simulink model "cIPC_l2originalLoad"  (R2024b)
settings: Solver=FixedStepDiscrete  StartTime=0.0  StopTime=TMax  FixedStep=DT  RelTol=1e-3
undefined symbols (not defined in the file): DiscIntNeverNeededParam, DT, Ki, optimal_azimuth_offset_rad
libraries: simulink_extras x1
settings Model: Creator=jhummel  LastModifiedBy=jhummel
settings ModelReferenceCC: EnableRefExpFcnMdlSchedulingChecks=on
settings RTWCC: GPUComputeCapability=3.5

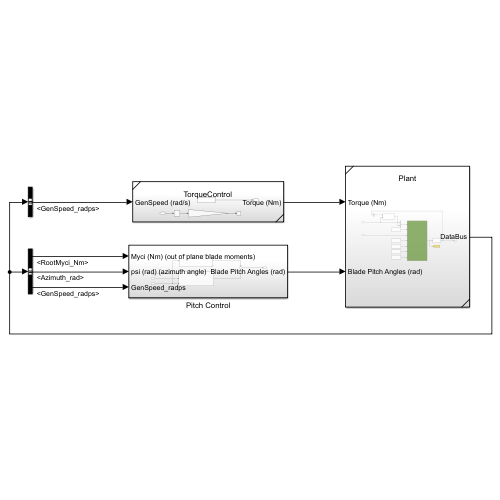
[thumbnail: Simulink's stored preview of the top-level diagram]
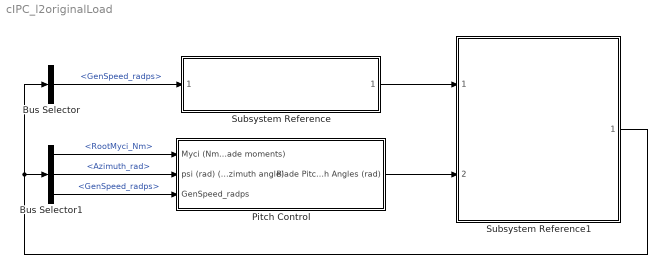
== system cIPC_l2originalLoad ==
  Bus Selector : BusSelector  OutputSignals=GenSpeed_radps
  Bus Selector1 : BusSelector  OutputSignals=RootMyci_Nm,Azimuth_rad,GenSpeed_radps
  Pitch Control : Subsystem
  Subsystem Reference : Subsystem  ReferencedSubsystem=TorqueControl
  Subsystem Reference1 : Subsystem  ReferencedSubsystem=Plant
  wires:
  Bus Selector/1 -> Subsystem Reference/1  "<GenSpeed_radps>"
  Bus Selector1/1 -> Pitch Control/1(Myci (Nm) (out of plane blade moments))  "<RootMyci_Nm>"
  Bus Selector1/2 -> Pitch Control/2(psi (rad) (azimuth angle))  "<Azimuth_rad>"
  Bus Selector1/3 -> Pitch Control/3(GenSpeed_radps)  "<GenSpeed_radps>"
  Subsystem Reference1/1 -> Bus Selector/1, Bus Selector1/1
  Pitch Control/1(Blade Pitch Angles (rad)) -> Subsystem Reference1/2
  Subsystem Reference/1 -> Subsystem Reference1/1

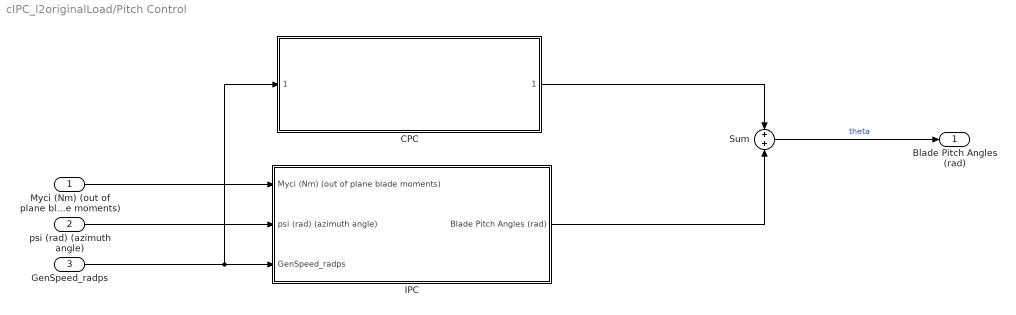
== system cIPC_l2originalLoad/Pitch Control ==
  Myci (Nm) (out of plane blade moments) : Inport
  psi (rad) (azimuth angle) : Inport  Port=2
  GenSpeed_radps : Inport  Port=3
  CPC : Subsystem  ReferencedSubsystem=CollectivePitchControl
  IPC : Subsystem
  Sum : Sum  Inputs=+|+
  Blade Pitch Angles (rad) : Outport
  wires:
  Myci (Nm) (out of plane blade moments)/1 -> IPC/1(Myci (Nm) (out of plane blade moments))
  psi (rad) (azimuth angle)/1 -> IPC/2(psi (rad) (azimuth angle))
  GenSpeed_radps/1 -> CPC/1, IPC/3(GenSpeed_radps)
  CPC/1 -> Sum/1
  Sum/1 -> Blade Pitch Angles (rad)/1  "theta"
  IPC/1(Blade Pitch Angles (rad)) -> Sum/2

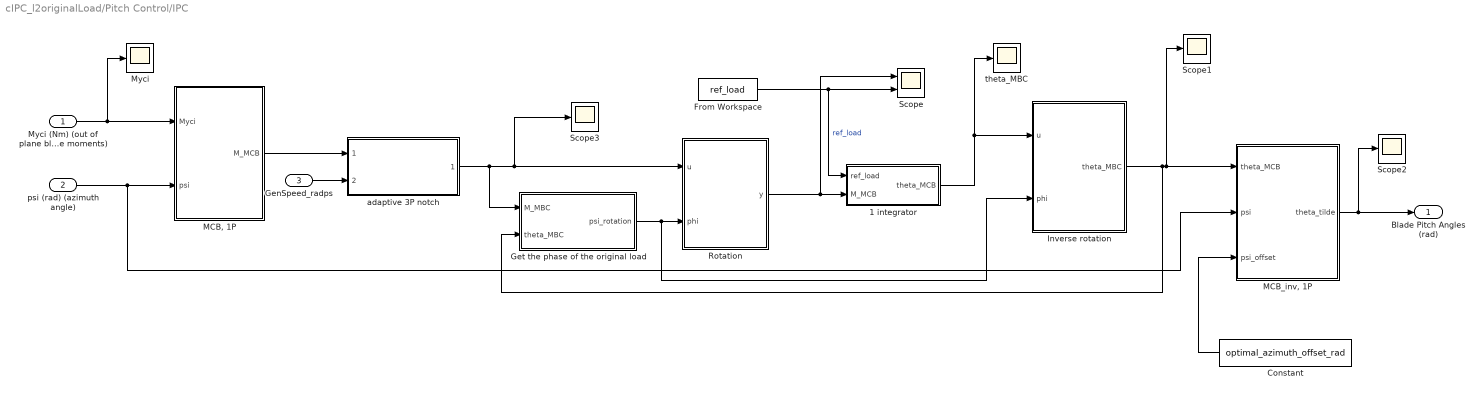
== system cIPC_l2originalLoad/Pitch Control/IPC ==
  Myci (Nm) (out of plane blade moments) : Inport
  psi (rad) (azimuth angle) : Inport  Port=2
  GenSpeed_radps : Inport  Port=3
  1 integrator : Subsystem
  Constant : Constant  Value=optimal_azimuth_offset_rad
  From Workspace : FromWorkspace  VariableName=ref_load  SampleTime=DT
  Get the phase of the original load : Subsystem
  Inverse rotation : Subsystem
  "MCB, 1P" : MATLAB Function  TreatAsAtomicUnit=on
  "MCB_inv, 1P" : MATLAB Function  TreatAsAtomicUnit=on
  Myci : Scope
  Rotation : MATLAB Function  TreatAsAtomicUnit=on
  Scope : Scope  NumInputPorts=2
  Scope1 : Scope
  Scope2 : Scope
  Scope3 : Scope
  adaptive 3P notch : Subsystem  ReferencedSubsystem=LoadFilter
  theta_MBC : Scope
  Blade Pitch Angles (rad) : Outport
  wires:
  Constant/1 -> "MCB_inv, 1P"/3(psi_offset)
  Myci (Nm) (out of plane blade moments)/1 -> "MCB, 1P"/1(Myci), Myci/1
  GenSpeed_radps/1 -> adaptive 3P notch/2
  psi (rad) (azimuth angle)/1 -> "MCB_inv, 1P"/2(psi), "MCB, 1P"/2(psi)
  Rotation/1(y) -> Scope/1, 1 integrator/2(M_MCB)
  1 integrator/1(theta_MCB) -> theta_MBC/1, Inverse rotation/1(u)
  adaptive 3P notch/1 -> Scope3/1, Rotation/1(u), Get the phase of the original load/1(M_MBC)
  From Workspace/1 -> 1 integrator/1(ref_load), Scope/2  "ref_load"
  Get the phase of the original load/1(psi_rotation) -> Inverse rotation/2(phi), Rotation/2(phi)
  "MCB_inv, 1P"/1(theta_tilde) -> Blade Pitch Angles (rad)/1, Scope2/1
  Inverse rotation/1(theta_MBC) -> Get the phase of the original load/2(theta_MBC), Scope1/1, "MCB_inv, 1P"/1(theta_MCB)
  "MCB, 1P"/1(M_MCB) -> adaptive 3P notch/1

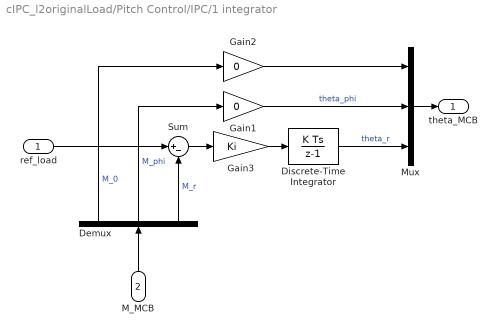
== system cIPC_l2originalLoad/Pitch Control/IPC/1 integrator ==
  ref_load : Inport
  M_MCB : Inport  Port=2
  Demux : Demux  Outputs=3
  Discrete-Time Integrator : DiscreteIntegrator  gainval=1  SampleTime=-1  LimitOutput=on  LowerSaturationLimit=0  ICPrevOutput=DiscIntNeverNeededParam  ICPrevScaledInput=DiscIntNeverNeededParam
  Gain1 : Gain  Gain=0
  Gain2 : Gain  Gain=0
  Gain3 : Gain  Gain=Ki
  Mux : Mux  Inputs=3
  Sum : Sum  Inputs=|+-
  theta_MCB : Outport
  wires:
  M_MCB/1 -> Demux/1
  Demux/2 -> Gain1/1  "M_phi"
  Demux/1 -> Gain2/1  "M_0"
  Mux/1 -> theta_MCB/1
  Gain1/1 -> Mux/2  "theta_phi"
  Gain2/1 -> Mux/1
  Discrete-Time Integrator/1 -> Mux/3  "theta_r"
  Sum/1 -> Gain3/1
  Gain3/1 -> Discrete-Time Integrator/1
  Demux/3 -> Sum/2  "M_r"
  ref_load/1 -> Sum/1

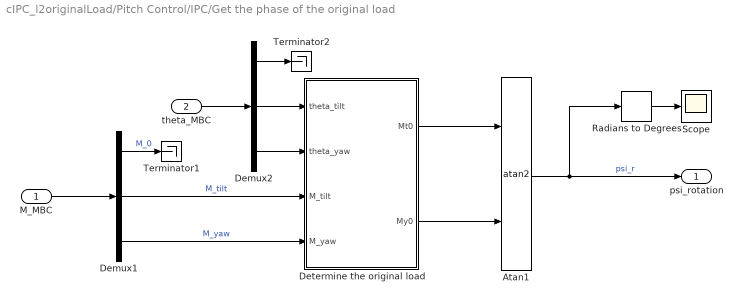
== system cIPC_l2originalLoad/Pitch Control/IPC/Get the phase of the original load ==
  M_MBC : Inport
  theta_MBC : Inport  Port=2
  Atan1 : Trigonometry  Operator=atan2
  Demux1 : Demux  Outputs=3
  Demux2 : Demux  Outputs=3
  Determine the original load : Subsystem
  Radians to Degrees : simulink_extras/Transformations/Radians to Degrees
  Scope : Scope
  Terminator1 : Terminator
  Terminator2 : Terminator
  psi_rotation : Outport
  wires:
  Demux1/3 -> Determine the original load/4(M_yaw)  "M_yaw"
  Demux1/1 -> Terminator1/1  "M_0"
  Demux1/2 -> Determine the original load/3(M_tilt)  "M_tilt"
  M_MBC/1 -> Demux1/1
  Atan1/1 -> psi_rotation/1, Radians to Degrees/1  "psi_r"
  Demux2/2 -> Determine the original load/1(theta_tilt)
  Demux2/3 -> Determine the original load/2(theta_yaw)
  theta_MBC/1 -> Demux2/1
  Demux2/1 -> Terminator2/1
  Determine the original load/2(My0) -> Atan1/2
  Determine the original load/1(Mt0) -> Atan1/1
  Radians to Degrees/1 -> Scope/1

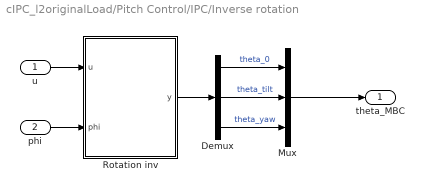
== system cIPC_l2originalLoad/Pitch Control/IPC/Inverse rotation ==
  u : Inport
  phi : Inport  Port=2
  Demux : Demux  Outputs=3
  Mux : Mux  Inputs=3
  Rotation inv : MATLAB Function  TreatAsAtomicUnit=on
  theta_MBC : Outport
  wires:
  Demux/1 -> Mux/1  "theta_0"
  Rotation inv/1(y) -> Demux/1
  Mux/1 -> theta_MBC/1
  u/1 -> Rotation inv/1(u)
  Demux/2 -> Mux/2  "theta_tilt"
  phi/1 -> Rotation inv/2(phi)
  Demux/3 -> Mux/3  "theta_yaw"

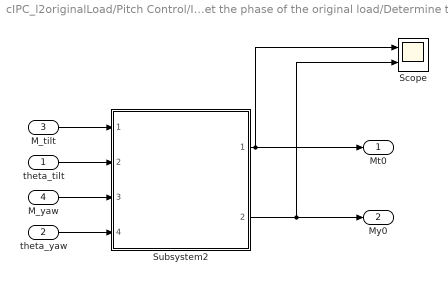
== system cIPC_l2originalLoad/Pitch Control/IPC/Get the phase of the original load/Determine the original load ==
  theta_tilt : Inport
  theta_yaw : Inport  Port=2
  M_tilt : Inport  Port=3
  M_yaw : Inport  Port=4
  Scope : Scope  NumInputPorts=2
  Subsystem2 : Subsystem  ReferencedSubsystem=OriginalLoadsEstimator
  Mt0 : Outport
  My0 : Outport  Port=2
  wires:
  Subsystem2/2 -> Scope/2, My0/1
  Subsystem2/1 -> Scope/1, Mt0/1
  M_tilt/1 -> Subsystem2/1
  theta_tilt/1 -> Subsystem2/2
  M_yaw/1 -> Subsystem2/3
  theta_yaw/1 -> Subsystem2/4

== matlab function cIPC_l2originalLoad/Pitch Control/IPC/MCB_inv, 1P ==
  data: theta_MCB input; theta_tilde output; psi input; psi_offset input
function theta_tilde = fcn(theta_MCB, psi, psi_offset)

theta_tilde = MBC_inv(theta_MCB, psi, psi_offset, 3, 1);

end

== matlab function cIPC_l2originalLoad/Pitch Control/IPC/MCB, 1P ==
  data: Myci input; M_MCB output; psi input
function M_MCB = fcn(Myci, psi)

% Do the coordinate transformation.
M_MCB = MBC(Myci, psi, 0, 3, 1);

end

== matlab function cIPC_l2originalLoad/Pitch Control/IPC/Rotation ==
  data: u input; y output; phi input
function y = fcn(u, phi)
% Rotate the vector u with the angle phi.
% This is a CCW rotation matrix, but since we're operating in a left-handed
% coordinate system, this will result in a CW rotation of the load to the
% yaw axis, now called the _r axis.

% Allocate space.
y = zeros(size(u));

R = [1,        0,         0;
     0, cos(phi), -sin(phi);
     0, sin(phi),  cos(phi)];

y = R * u;

end

== matlab function cIPC_l2originalLoad/Pitch Control/IPC/Inverse rotation/Rotation inv ==
  data: u input; y output; phi input
function y = fcn(u, phi)
% Rotate the vector u with the angle phi.
% This is a CW rotation matrix. But since we're operating in a left-handed
% coordinate system it results in a CCW rotation.

% Allocate space.
y = zeros(size(u));

R = [1,         0,        0;
     0,  cos(phi), sin(phi);
     0, -sin(phi), cos(phi)];

y = R * u;

end
